simulink model "WindTunnel2"  (R2016b)
settings: Solver=VariableStepAuto  StartTime=0.0  StopTime=20  MaxStep=0.01  RelTol=1e-3
undefined symbols (not defined in the file or in its folder): P, Scale2
libraries: simulink x12
settings Model: Creator=CFRPG  LastModifiedBy=CFRPG

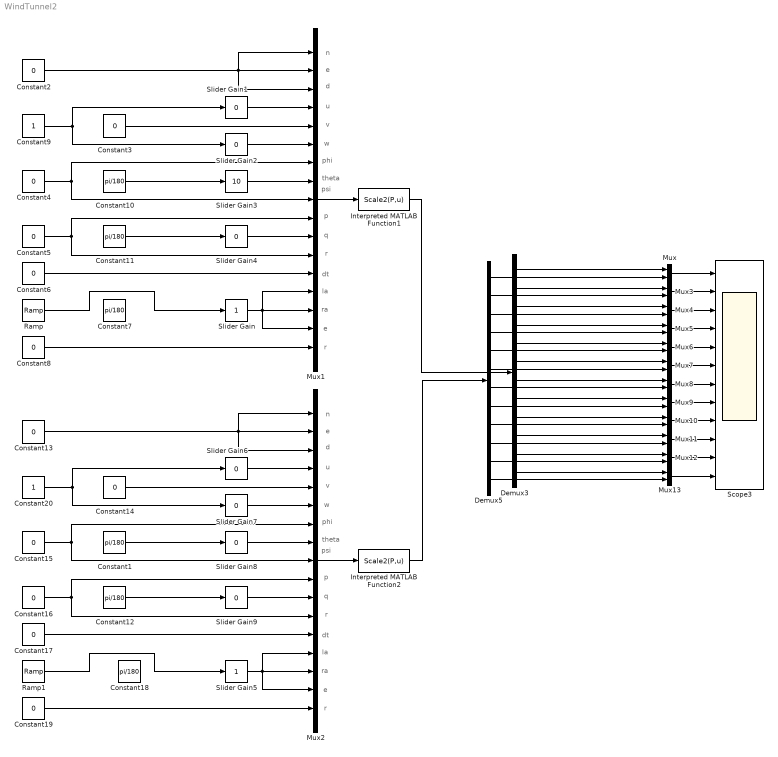
== system WindTunnel2 ==
  note: r
  note: e
  note: ra
  note: la
  note: dt
  note: r
  note: q
  note: p
  note: psi
  note: theta
  note: phi
  note: w
  note: v
  note: u
  note: d
  note: e
  note: n
  note: r
  note: e
  note: ra
  note: la
  note: dt
  note: r
  note: q
  note: p
  note: psi
  note: theta
  note: phi
  note: w
  note: v
  note: u
  note: d
  note: e
  note: n
  Constant{1,7,10..12,18} (6 alike) : Constant  Value=pi/180
  Constant{2..6,8,13..17,19} (12 alike) : Constant  Value=0
  Constant20 : Constant
  Constant9 : Constant
  Demux3 : Demux  Outputs=12
  Demux5 : Demux  Outputs=12
  Interpreted MATLAB Function1 : MATLABFcn  MATLABFcn=Scale2(P,u)
  Interpreted MATLAB Function2 : MATLABFcn  MATLABFcn=Scale2(P,u)
  Mux{,3..13} (12 alike) : Mux  Inputs=2
  Mux1 : Mux  Inputs=17
  Mux2 : Mux  Inputs=17
  Ramp : simulink/Sources/Ramp  slope=pi/10  start=0  X0=0
  Ramp1 : simulink/Sources/Ramp  slope=pi/10  start=0  X0=0
  Scope3 : Scope  NumInputPorts=12
  Slider Gain : simulink/Math Operations/Slider Gain  low=-360  gain=1  high=360
  Slider Gain1 : simulink/Math Operations/Slider Gain  low=0  gain=0  high=20
  Slider Gain2 : simulink/Math Operations/Slider Gain  low=-20  gain=0  high=20
  Slider Gain3 : simulink/Math Operations/Slider Gain  low=-360  gain=10  high=360
  Slider Gain4 : simulink/Math Operations/Slider Gain  low=-360  gain=0  high=360
  Slider Gain5 : simulink/Math Operations/Slider Gain  low=-360  gain=1  high=360
  Slider Gain6 : simulink/Math Operations/Slider Gain  low=0  gain=0  high=20
  Slider Gain7 : simulink/Math Operations/Slider Gain  low=-20  gain=0  high=20
  Slider Gain8 : simulink/Math Operations/Slider Gain  low=-360  gain=0  high=360
  Slider Gain9 : simulink/Math Operations/Slider Gain  low=-360  gain=0  high=360
  wires:
  Interpreted MATLAB Function1/1 -> Demux3/1
  Mux1/1 -> Interpreted MATLAB Function1/1
  Constant2/1 -> Mux1/3, Mux1/1, Mux1/2
  Constant3/1 -> Mux1/5
  Constant4/1 -> Mux1/9, Mux1/7
  Constant5/1 -> Mux1/10, Mux1/12
  Constant6/1 -> Mux1/13
  Slider Gain/1 -> Mux1/16, Mux1/15, Mux1/14
  Ramp/1 -> Slider Gain/1
  Constant8/1 -> Mux1/17
  Slider Gain1/1 -> Mux1/4
  Slider Gain2/1 -> Mux1/6
  Constant9/1 -> Slider Gain2/1, Slider Gain1/1
  Slider Gain3/1 -> Mux1/8
  Constant10/1 -> Slider Gain3/1
  Constant11/1 -> Slider Gain4/1
  Slider Gain4/1 -> Mux1/11
  Interpreted MATLAB Function2/1 -> Demux5/1
  Mux2/1 -> Interpreted MATLAB Function2/1
  Constant13/1 -> Mux2/3, Mux2/1, Mux2/2
  Constant14/1 -> Mux2/5
  Constant15/1 -> Mux2/9, Mux2/7
  Constant16/1 -> Mux2/10, Mux2/12
  Constant17/1 -> Mux2/13
  Slider Gain5/1 -> Mux2/16, Mux2/15, Mux2/14
  Ramp1/1 -> Slider Gain5/1
  Constant19/1 -> Mux2/17
  Slider Gain6/1 -> Mux2/4
  Slider Gain7/1 -> Mux2/6
  Constant20/1 -> Slider Gain7/1, Slider Gain6/1
  Slider Gain8/1 -> Mux2/8
  Constant1/1 -> Slider Gain8/1
  Constant12/1 -> Slider Gain9/1
  Slider Gain9/1 -> Mux2/11
  Demux3/1 -> Mux/1
  Demux3/2 -> Mux3/1
  Demux3/3 -> Mux4/1
  Demux3/4 -> Mux5/1
  Demux3/5 -> Mux6/1
  Demux3/6 -> Mux7/1
  Demux3/7 -> Mux8/1
  Demux3/8 -> Mux9/1
  Demux3/9 -> Mux10/1
  Demux3/10 -> Mux11/1
  Demux3/11 -> Mux12/1
  Demux3/12 -> Mux13/1
  Demux5/1 -> Mux/2
  Demux5/2 -> Mux3/2
  Demux5/3 -> Mux4/2
  Demux5/4 -> Mux5/2
  Demux5/5 -> Mux6/2
  Demux5/6 -> Mux7/2
  Demux5/7 -> Mux8/2
  Demux5/8 -> Mux9/2
  Demux5/9 -> Mux10/2
  Demux5/10 -> Mux11/2
  Demux5/11 -> Mux12/2
  Demux5/12 -> Mux13/2
  Mux/1 -> Scope3/1
  Mux3/1 -> Scope3/2
  Mux4/1 -> Scope3/3
  Mux5/1 -> Scope3/4
  Mux6/1 -> Scope3/5
  Mux7/1 -> Scope3/6
  Mux8/1 -> Scope3/7
  Mux9/1 -> Scope3/8
  Mux10/1 -> Scope3/9
  Mux11/1 -> Scope3/10
  Mux12/1 -> Scope3/11
  Mux13/1 -> Scope3/12
